simulink model "inrush"  (R2016b)
settings: Solver=FixedStepDiscrete  StartTime=0.0  StopTime=1  FixedStep=1/2400  RelTol=1e-3
libraries: powerlib x12, utilities x6
settings Model: Creator=bclzl  LastModifiedBy=bclzl
settings DebuggingCC: UnconnectedInputMsg=none  UnconnectedOutputMsg=none  UnconnectedLineMsg=none

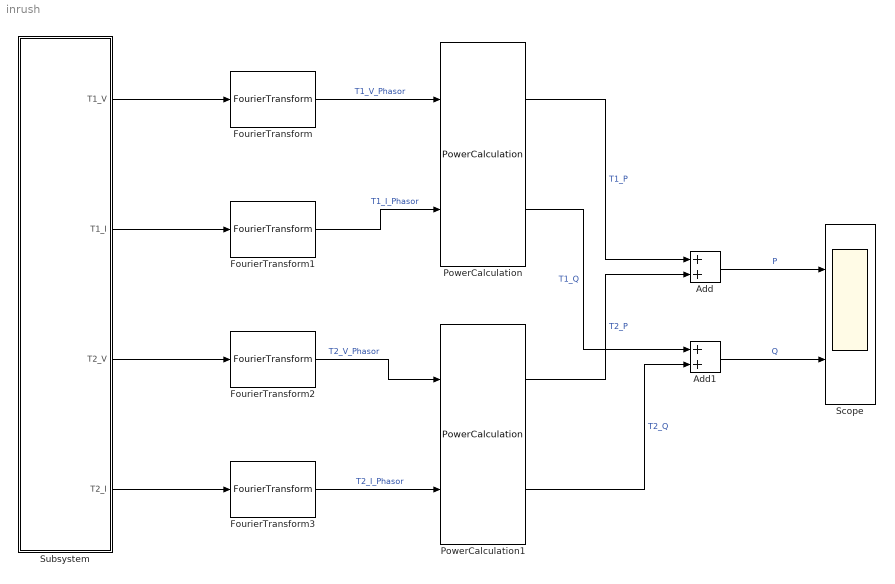
== system inrush ==
  Add : Sum
  Add1 : Sum
  FourierTransform{,1..3} (4 alike) : utilities/FourierTransform
  PowerCalculation : utilities/PowerCalculation
  PowerCalculation1 : utilities/PowerCalculation
  Scope : Scope  NumInputPorts=2
  Subsystem : Subsystem
  wires:
  Subsystem/2(T1_I) -> FourierTransform1/1
  Subsystem/1(T1_V) -> FourierTransform/1
  FourierTransform/1 -> PowerCalculation/1  "T1_V_Phasor"
  FourierTransform1/1 -> PowerCalculation/2  "T1_I_Phasor"
  PowerCalculation/1 -> Add/1  "T1_P"
  PowerCalculation/2 -> Add1/1  "T1_Q"
  Subsystem/3(T2_V) -> FourierTransform2/1
  Subsystem/4(T2_I) -> FourierTransform3/1
  FourierTransform3/1 -> PowerCalculation1/2  "T2_I_Phasor"
  FourierTransform2/1 -> PowerCalculation1/1  "T2_V_Phasor"
  Add/1 -> Scope/1  "P"
  Add1/1 -> Scope/2  "Q"
  PowerCalculation1/1 -> Add/2  "T2_P"
  PowerCalculation1/2 -> Add1/2  "T2_Q"

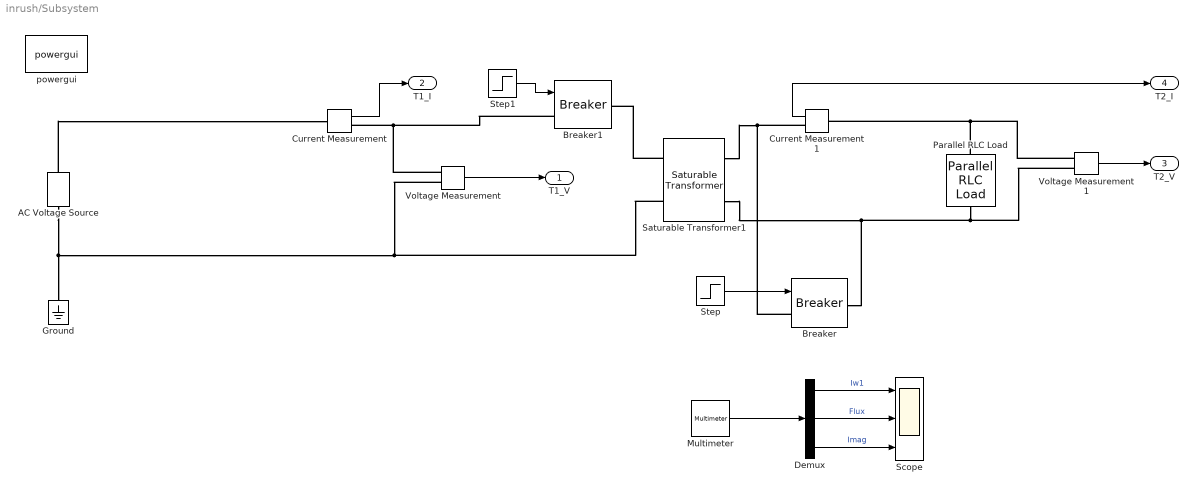
== system inrush/Subsystem ==
  AC Voltage Source : powerlib/Electrical Sources/AC Voltage Source  Amplitude=735000*sqrt(2)  Phase=0  Frequency=50  SampleTime=0  Measurements=None  BusType=PV  Pref=10e3  Qref=0  Qmin=-inf  Qmax=+inf
  Breaker : powerlib/Elements/Breaker  InitialState=0  SwitchingTimes="[1/60  5/60]"  External=on  BreakerResistance=0.01  SnubberResistance=1e6  SnubberCapacitance=inf  Measurements=None  MoreParameters=on  NoBreakLoop=off
  Breaker1 : powerlib/Elements/Breaker  InitialState=0  SwitchingTimes="[1/60  5/60]"  External=on  BreakerResistance=0.01  SnubberResistance=1e6  SnubberCapacitance=inf  Measurements=None  MoreParameters=on  NoBreakLoop=off
  Current Measurement : powerlib/Measurements/Current Measurement  PhasorSimulation=off  OutputType=Complex  PSBequivalent=0
  Current Measurement1 : powerlib/Measurements/Current Measurement  PhasorSimulation=off  OutputType=Complex  PSBequivalent=0
  Demux : Demux  Outputs=3
  Ground : powerlib/Elements/Ground  LConnTagsString=a
  Multimeter : powerlib/Measurements/Multimeter  PhasorSimulation=off  OutputType=Complex  sel=[3 7 6]  L=7  Gain=[1 1 1]  yselected={'Iw1: Subsystem/Saturable Transformer1','Flux: Subsystem/Saturable Transformer1','Imag: Subsystem/Saturable Transformer1'};  PSBOutputType=1  PSBequivalent=0  AxesSetting=[0,0.1,-100,100]  Display=0  SavedBlockNames=-11
  Parallel RLC Load : powerlib/Elements/Parallel RLC Load  LConnTagsString=a  RConnTagsString=__new0  NominalVoltage=315000  NominalFrequency=50  ActivePower=10e3  InductivePower=100  CapacitivePower=100  Setx0=on  InitialVoltage=0  SetiL0=on  InitialCurrent=0  Measurements=None  LoadType=constant Z
      settings: AttributesFormatString=\n
  Saturable Transformer1 : powerlib/Elements/Saturable Transformer  ThreeWindings=off  Hysteresis=off  DataFile='hysteresis.mat'  Measurements=All measurements (V I Flux)  UNITS=pu  NominalPower=[250e6 50]  Winding1="[ 735e3  0.002  0.08 ]"  Winding2="[ 315e3  0.002  0.08 ]"  Winding3="[ 315e3  0.002  0.08 ]"  Saturation=[ 0,0 ; 0.5,1.1; 1.0,1.2 ; 1.2,1.52 ]  CoreLoss=[500 0]  MoreParameters=off  BreakLoop=off  DataType=off  InitialFlux=-1555.01133110333  TransfoNumber=1
  Scope : Scope  NumInputPorts=3
  Step : Step  Time=1.5  SampleTime=0
  Step1 : Step  Time=0  SampleTime=0
  Voltage Measurement : powerlib/Measurements/Voltage Measurement  PhasorSimulation=off  OutputType=Complex  PSBequivalent=0
  Voltage Measurement1 : powerlib/Measurements/Voltage Measurement  PhasorSimulation=off  OutputType=Complex  PSBequivalent=0
  powergui : powerlib/powergui  Priority=1  SimulationMode=Discrete  SolverType=Tustin/Backward Euler (TBE)  SampleTime=1/2400  frequency=60  SPID=on  DisableSnubberDevices=on  DisableRonSwitches=on  DisableVfSwitches=on  SwTol=0  DisplayEquations=on  Interpol=off  ExternalGateDelay=off  methode=off  Ts=10  FunctionMessages=off  echomessages=off  HookPort=off  EnableUseOfTLC=off  x0status=zero  frequencyindice=50  Pbase=100e6  ErrMax=1e-4  Iterations=50  UnitsV=kV  UnitsW=MW  buscounter=0  RestoreLinks=warning  ResistiveCurrentMeasurement=off  Frange=[0:2:500]  Ylog=off  Xlog=on  ShowGrid=off  save=off  variable=ZData  structure=0  ZoomFFT=off  StartTime=0.0  cycles=1  DisplayStyle=1  fundamental=60  FreqAxis=off  MaxFrequency=1000  frequencyindicesteady=1  RmsSteady=1  display=off
  T1_V : Outport
  T1_I : Outport  Port=2
  T2_V : Outport  Port=3
  T2_I : Outport  Port=4
  wires:
  Voltage Measurement1/1 -> T2_V/1
  Current Measurement1/1 -> T2_I/1
  Step/1 -> Breaker/1
  Step1/1 -> Breaker1/1
  Current Measurement/1 -> T1_I/1
  Voltage Measurement/1 -> T1_V/1
  Multimeter/1 -> Demux/1
  Demux/2 -> Scope/2  "Flux"
  Demux/1 -> Scope/1  "Iw1"
  Demux/3 -> Scope/3  "Imag"
  connections:
  AC Voltage Source/RConn1 -- Current Measurement/LConn1
  Voltage Measurement/LConn1 -- Breaker1/LConn1 -- Current Measurement/RConn1
  Parallel RLC Load/RConn1 -- Voltage Measurement1/LConn2 -- Saturable Transformer1/RConn2 -- Breaker/RConn1
  Parallel RLC Load/LConn1 -- Voltage Measurement1/LConn1 -- Current Measurement1/LConn1
  Current Measurement1/RConn1 -- Saturable Transformer1/RConn1 -- Breaker/LConn1
  Saturable Transformer1/LConn1 -- Breaker1/RConn1
  AC Voltage Source/LConn1 -- Saturable Transformer1/LConn2 -- Voltage Measurement/LConn2 -- Ground/LConn1
